simulink model "TF_Simulations"  (R2018a)
settings: Solver=VariableStepAuto  StartTime=0.0  StopTime=6  RelTol=1e-3
settings Model: Creator=yakhti  LastModifiedBy=yakhti

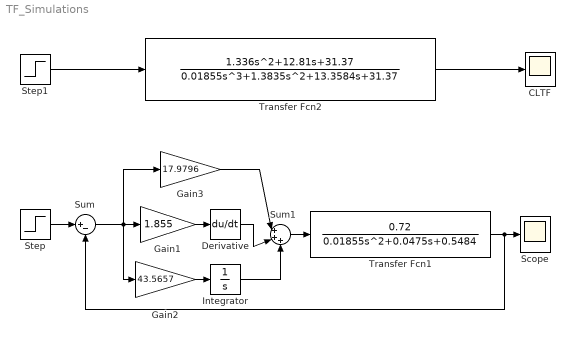
== system TF_Simulations ==
  CLTF : Scope
  Derivative : Derivative
  Gain1 : Gain  Gain=1.855
  Gain2 : Gain  Gain=43.5657
  Gain3 : Gain  Gain=17.9796
  Integrator : Integrator
  Scope : Scope
  Step : Step  Time=0  SampleTime=0
  Step1 : Step  Time=0  SampleTime=0
  Sum : Sum  Inputs=|+-
  Sum1 : Sum  Inputs=|+++
  Transfer Fcn1 : TransferFcn  Numerator=[0.72]  Denominator=[0.01855 0.0475 0.5484]
  Transfer Fcn2 : TransferFcn  Numerator=[1.336 12.81 31.37]  Denominator=[0.01855 1.3835 13.3584 31.37]
  wires:
  Transfer Fcn2/1 -> CLTF/1
  Sum1/1 -> Transfer Fcn1/1
  Step/1 -> Sum/1
  Step1/1 -> Transfer Fcn2/1
  Transfer Fcn1/1 -> Sum/2, Scope/1
  Gain3/1 -> Sum1/1
  Derivative/1 -> Sum1/2
  Integrator/1 -> Sum1/3
  Gain2/1 -> Integrator/1
  Gain1/1 -> Derivative/1
  Sum/1 -> Gain1/1, Gain3/1, Gain2/1
